simulink model "jifenjiaozheng1"  (R2022b)
settings: Solver=VariableStepAuto  StartTime=0.0  StopTime=20  RelTol=1e-3
settings Model: Creator=HONOR  LastModifiedBy=acer
settings DebuggingCC: UnconnectedInputMsg=warning  UnconnectedOutputMsg=warning  UnconnectedLineMsg=warning
settings ModelReferenceCC: EnableRefExpFcnMdlSchedulingChecks=on
settings RTWCC: DLArmComputeVersion=19.05

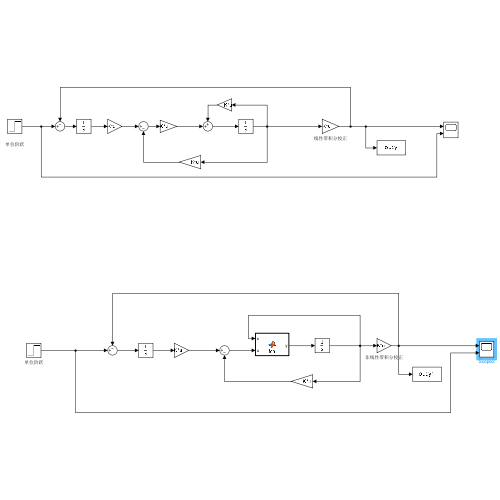
[thumbnail: Simulink's stored preview of the top-level diagram]
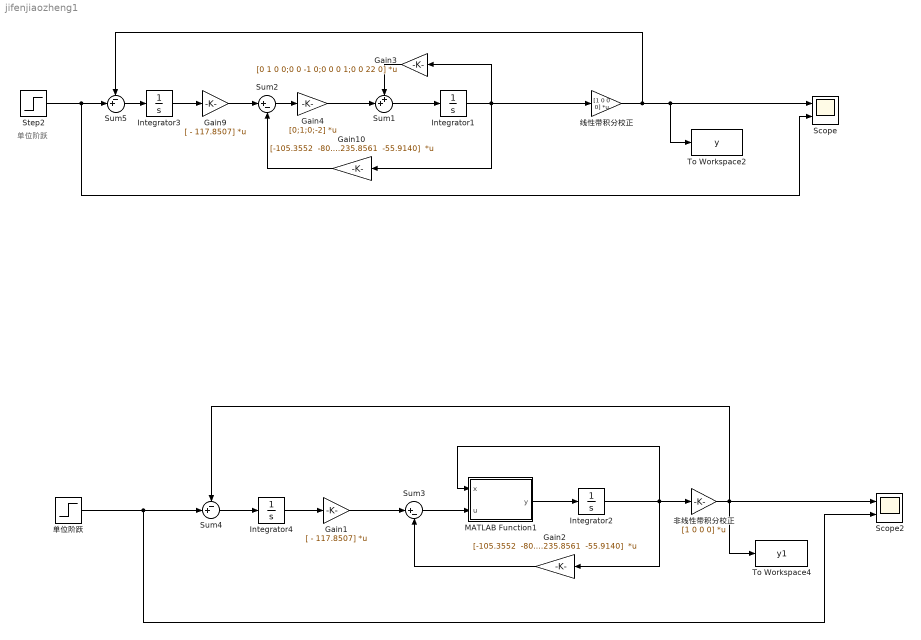
== system jifenjiaozheng1 ==
  note: 单位阶跃
  Gain1 : Gain  Gain=[ - 117.8507]  Multiplication=Matrix(K*u)
  Gain10 : Gain  Gain="[-105.3552  -80.4281 -235.8561  -55.9140]"  Multiplication=Matrix(K*u)
  Gain2 : Gain  Gain="[-105.3552  -80.4281 -235.8561  -55.9140]"  Multiplication=Matrix(K*u)
  Gain3 : Gain  Gain=[0 1 0 0;0 0 -1 0;0 0 0 1;0 0 22 0]  Multiplication=Matrix(K*u)
  Gain4 : Gain  Gain=[0;1;0;-2]  Multiplication=Matrix(K*u)
  Gain9 : Gain  Gain=[ - 117.8507]  Multiplication=Matrix(K*u)
  Integrator1 : Integrator  InitialCondition=[0,0,0.1,0]
  Integrator2 : Integrator  InitialCondition=[0,0,0.1,0]
  Integrator3 : Integrator  InitialCondition=[0]
  Integrator4 : Integrator  InitialCondition=[0]
  MATLAB Function1 : MATLAB Function  TreatAsAtomicUnit=on
  Scope : Scope  NumInputPorts=2
  Scope2 : Scope  NumInputPorts=2
  Step2 : Step  SampleTime=0
  Sum1 : Sum  Inputs=++|
  Sum2 : Sum  Inputs=|+-
  Sum3 : Sum  Inputs=|+-
  Sum4 : Sum  Inputs=-+|
  Sum5 : Sum  Inputs=-+|
  To Workspace2 : ToWorkspace  VariableName=y  SaveFormat=Structure With Time  SampleTime=-1
  To Workspace4 : ToWorkspace  VariableName=y1  SaveFormat=Structure With Time  SampleTime=-1
  单位阶跃 : Step  SampleTime=0
  线性带积分校正 : Gain  Gain=[1 0 0 0]  Multiplication=Matrix(K*u)
  非线性带积分校正 : Gain  Gain=[1 0 0 0]  Multiplication=Matrix(K*u)
  wires:
  Integrator1/1 -> Gain10/1, 线性带积分校正/1, Gain3/1
  Gain9/1 -> Sum2/1
  Sum1/1 -> Integrator1/1
  Sum2/1 -> Gain4/1
  Gain4/1 -> Sum1/2
  Gain3/1 -> Sum1/1
  线性带积分校正/1 -> To Workspace2/1, Scope/1, Sum5/1
  Sum5/1 -> Integrator3/1
  Step2/1 -> Scope/2, Sum5/2
  Integrator3/1 -> Gain9/1
  Gain10/1 -> Sum2/2
  Integrator2/1 -> Gain2/1, MATLAB Function1/1(x), 非线性带积分校正/1
  MATLAB Function1/1(y) -> Integrator2/1
  Integrator4/1 -> Gain1/1
  Sum3/1 -> MATLAB Function1/2(u)
  非线性带积分校正/1 -> Sum4/1, Scope2/1, To Workspace4/1
  单位阶跃/1 -> Scope2/2, Sum4/2
  Sum4/1 -> Integrator4/1
  Gain2/1 -> Sum3/2
  Gain1/1 -> Sum3/1

== matlab function jifenjiaozheng1/MATLAB Function1 ==
  data: x input; u input; y output
function y = fcn(x, u)
M=1;
m=0.1;
l=0.5;
g=10;
Dx3=x(4);
Dx4=(u*cos(x(3))-(M+m)*g*sin(x(3))+m*l*sin(x(3))*cos(x(3)*x(4)))/(m*l*cos(x(3))*cos(x(3))-(M+m)*l);
Dx1=x(2);
Dx2=((u+m*l*sin(x(3)*x(4)*x(4))-m*g*cos(x(3))*sin(x(3)))/(M+m-m*cos(x(3))*cos(x(3))));
y=[Dx1;Dx2;Dx3;Dx4];
